simulink subsystem "ModelBasedArmKinematics"  (R2023a)
settings: Solver=VariableStepAuto  StartTime=0.0  StopTime=10.0  RelTol=1e-3
values from neighbouring files (symbols this model uses):
  alpha = zeros(1, nLink)    [JointControl_Params.m]
settings Model: Creator=Andy  LastModifiedBy=Andy
settings OptimizationCC: ReuseModelBlockBuffer=off
settings ModelReferenceCC: EnableRefExpFcnMdlSchedulingChecks=on

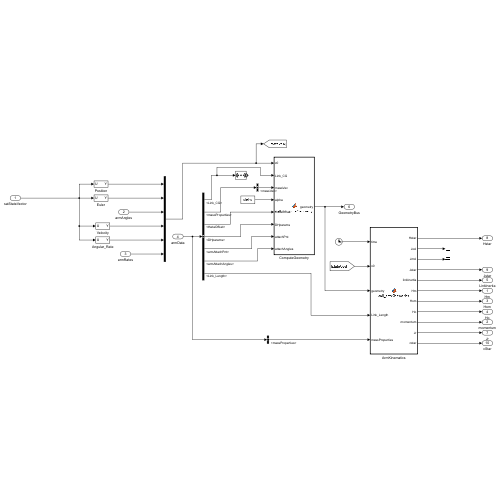
[thumbnail: Simulink's stored preview of the top-level diagram]
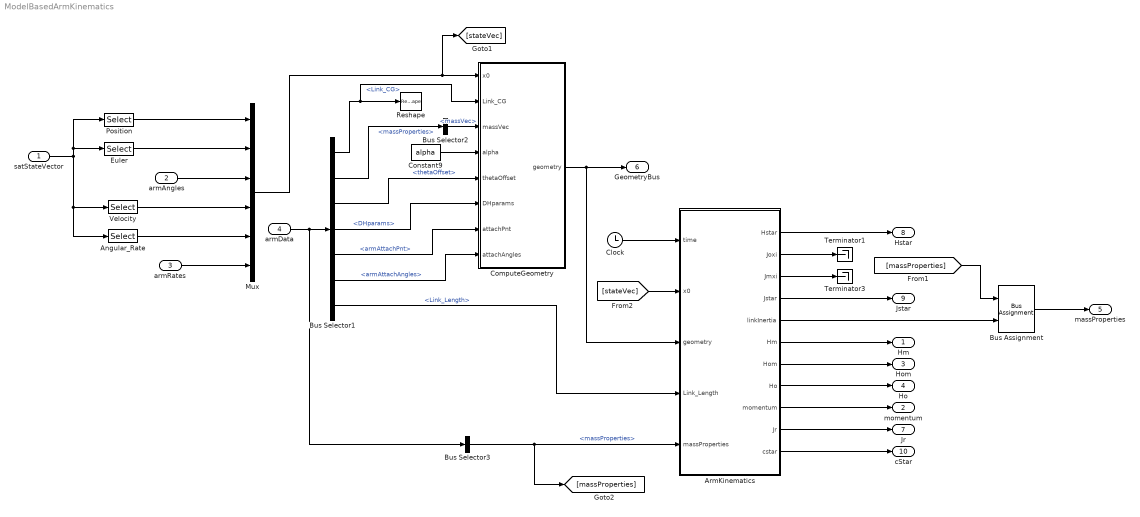
== system ModelBasedArmKinematics ==
  satStateVector : Inport
  armAngles : Inport  Port=2
  armRates : Inport  Port=3
  armData : Inport  Port=4
  Angular_Rate : Selector  InputPortWidth=12  IndexOptions=Index vector (dialog)  Indices=10:12  OutputSizes=1
  ArmKinematics : MATLAB Function
  Bus Assignment : BusAssignment  AssignedSignals=linkInertia
  Bus Selector1 : BusSelector  OutputSignals=Link_CG,massProperties,thetaOffset,DHparams,armAttachPnt,armAttachAngles,Link_Length
  Bus Selector2 : BusSelector  OutputSignals=massVec
  Bus Selector3 : BusSelector  OutputSignals=massProperties
  Clock : Clock
  ComputeGeometry : MATLAB Function
  Constant9 : Constant  Value=alpha
  Euler : Selector  InputPortWidth=12  IndexOptions=Index vector (dialog)  Indices=4:6  OutputSizes=1
  Mux : Mux  Inputs=6
  Position : Selector  InputPortWidth=12  IndexOptions=Index vector (dialog)  Indices=1:3  OutputSizes=1
  Reshape : Reshape  OutputDimensionality=Row vector (2-D)
  Terminator1 : Terminator
  Terminator3 : Terminator
  Velocity : Selector  InputPortWidth=12  IndexOptions=Index vector (dialog)  Indices=7:9  OutputSizes=1
  Hm : Outport
  momentum : Outport  Port=2
  Hom : Outport  Port=3
  Ho : Outport  Port=4
  massProperties : Outport  Port=5
  GeometryBus : Outport  Port=6
  Jr : Outport  Port=7
  Hstar : Outport  Port=8
  Jstar : Outport  Port=9
  cStar : Outport  Port=10
  wires:
  Bus Assignment/1 -> massProperties/1
  ArmKinematics/5(linkInertia) -> Bus Assignment/2
  [massProperties] -> Bus Assignment/1
  ArmKinematics/11(cstar) -> cStar/1
  Bus Selector3/1 -> ArmKinematics/5(massProperties), [massProperties]  "<massProperties>"
  Bus Selector2/1 -> ComputeGeometry/3(massVec)  "<massVec>"
  Bus Selector1/2 -> Bus Selector2/1  "<massProperties>"
  ArmKinematics/10(Jr) -> Jr/1
  ArmKinematics/4(Jstar) -> Jstar/1
  ArmKinematics/3(Jmxi) -> Terminator3/1
  ArmKinematics/2(Joxi) -> Terminator1/1
  ArmKinematics/8(Ho) -> Ho/1
  ArmKinematics/7(Hom) -> Hom/1
  ArmKinematics/9(momentum) -> momentum/1
  ArmKinematics/6(Hm) -> Hm/1
  ArmKinematics/1(Hstar) -> Hstar/1
  Bus Selector1/7 -> ArmKinematics/4(Link_Length)  "<Link_Length>"
  Bus Selector1/5 -> ComputeGeometry/7(attachPnt)  "<armAttachPnt>"
  Bus Selector1/4 -> ComputeGeometry/6(DHparams)  "<DHparams>"
  Bus Selector1/3 -> ComputeGeometry/5(thetaOffset)  "<thetaOffset>"
  Bus Selector1/1 -> ComputeGeometry/2(Link_CG), Reshape/1  "<Link_CG>"
  armData/1 -> Bus Selector3/1, Bus Selector1/1
  satStateVector/1 -> Position/1, Euler/1, Angular_Rate/1, Velocity/1
  Angular_Rate/1 -> Mux/5
  Velocity/1 -> Mux/4
  Euler/1 -> Mux/2
  Position/1 -> Mux/1
  armRates/1 -> Mux/6
  armAngles/1 -> Mux/3
  Mux/1 -> [stateVec], ComputeGeometry/1(x0)
  [stateVec] -> ArmKinematics/2(x0)
  Bus Selector1/6 -> ComputeGeometry/8(attachAngles)  "<armAttachAngles>"
  Clock/1 -> ArmKinematics/1(time)
  Constant9/1 -> ComputeGeometry/4(alpha)
  ComputeGeometry/1(geometry) -> GeometryBus/1, ArmKinematics/3(geometry)

== matlab function ModelBasedArmKinematics/ArmKinematics ==
  data: time input; Hstar output; Joxi output; Jmxi output; Jstar output; x0 input; geometry input Bus: GeometryBus; Link_Length input; massProperties input Bus: MassPropertiesBus; NLINKS parameter; linkInertia output; Hm output; Hom output; Ho output; momentum output; Jr output; cstar output
function [Hstar,Joxi,Jmxi,Jstar,linkInertia,Hm,Hom,Ho,momentum,Jr,cstar] = call_armKinematics(time,x0,geometry,Link_Length,massProperties,NLINKS)

nLink = NLINKS;

% Alias for joint angles and rates
jAngle = x0(7:7+nLink-1);
jRate  = x0(13+nLink:13+nLink+nLink-1);
qDot   = jRate';

% Compute components of the generalized inertia matrix
[Ho, Hom, Hsq, Hm, Hstar, HstarInv, HoInv, linkInertia, Jt, Jr] = computeMassMatrix(x0,geometry,massProperties,NLINKS);

% Compute the c star matrix
massProperties.linkInertia = linkInertia;
[cstar] = computeCstar(geometry,massProperties,jAngle,qDot,Jt,Jr,Hom,HoInv,Link_Length,NLINKS);

[Joxi,Jmxi,Jstar] = generalizedJacobian2(geometry,HoInv,Hom,NLINKS);

% Compute linear and angular momentum     
nState = size(x0,1);
momentum = Ho*x0(6+NLINKS+1:6+NLINKS+6) + Hom*x0(12+NLINKS+1:nState);

== matlab function ModelBasedArmKinematics/ComputeGeometry ==
  data: geometry output Bus: GeometryBus; x0 input; Link_CG input; massVec input; alpha input; thetaOffset input; DHparams input; attachPnt input; attachAngles input; NLINKS parameter
function geometry = call_computeGeometry(x0,Link_CG,massVec,alpha,thetaOffset,DHparams,attachPnt,attachAngles,NLINKS)

[geometry] = computeGeometry(x0,NLINKS,Link_CG,massVec,alpha,thetaOffset,DHparams,attachPnt,attachAngles);
